simulink model "Model_1"  (R2020b)
settings: Solver=VariableStepAuto  StartTime=0.0  StopTime=10.0  RelTol=1e-3
model workspace (MAT data in the model file):
  J = 3.2284e-06
  K = 0.0274
  L = 2.75e-06
  R = 4
  b = 3.5077e-06
settings Model: OrderedModelArguments=off  Creator=Diwakar Reddy  LastModifiedBy=Diwakar Reddy

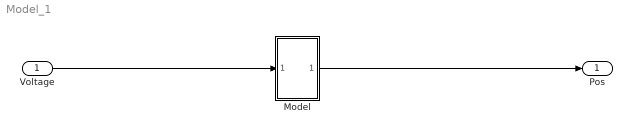
== system Model_1 ==
  Voltage : Inport
  Model : Subsystem
  Pos : Outport
  wires:
  Voltage/1 -> Model/1(In1)
  Model/1(Out1) -> Pos/1

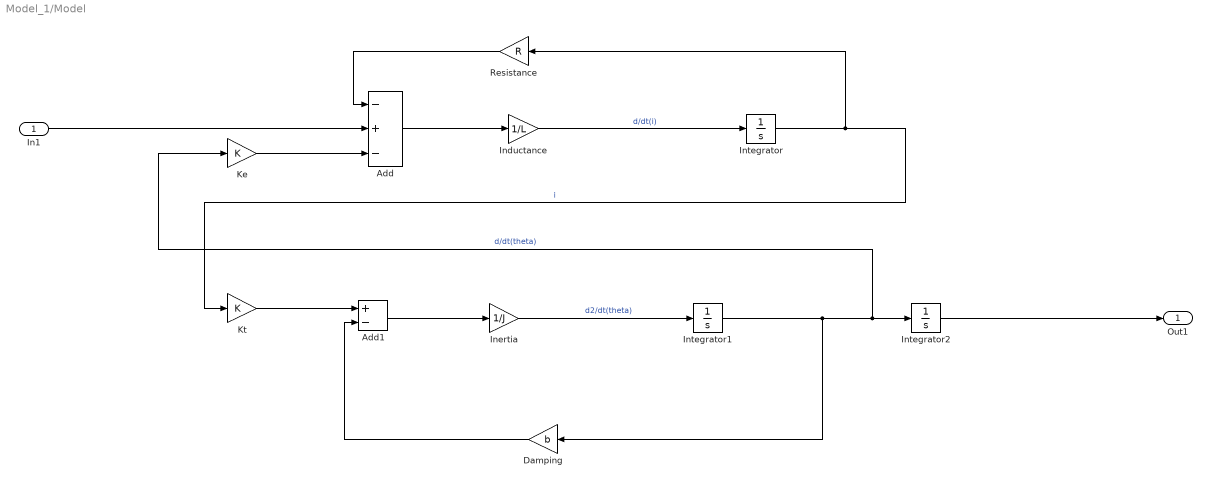
== system Model_1/Model ==
  In1 : Inport
  Add : Sum  Inputs=-+-
  Add1 : Sum  Inputs=+-
  Damping : Gain  Gain=b
  Inductance : Gain  Gain=1/L
  Inertia : Gain  Gain=1/J
  Integrator : Integrator
  Integrator1 : Integrator
  Integrator2 : Integrator
  Ke : Gain  Gain=K
  Kt : Gain  Gain=K
  Resistance : Gain  Gain=R
  Out1 : Outport
  wires:
  Resistance/1 -> Add/1
  Integrator1/1 -> Damping/1, Ke/1, Integrator2/1  "d/dt(theta)"
  Integrator/1 -> Resistance/1, Kt/1  "i"
  Inductance/1 -> Integrator/1  "d/dt(i)"
  Ke/1 -> Add/3
  In1/1 -> Add/2
  Add1/1 -> Inertia/1
  Integrator2/1 -> Out1/1
  Inertia/1 -> Integrator1/1  "d2/dt(theta)"
  Damping/1 -> Add1/2
  Kt/1 -> Add1/1
  Add/1 -> Inductance/1
